simulink model "trackingModel"  (R2020b)
settings: Solver=VariableStepAuto  StartTime=0.0  StopTime=1.0  FixedStep=(1/16367600)/3  RelTol=1e-3
values from neighbouring files (symbols this model uses):
  fcBasis = 4128460    [config.m]
  fs = 16367600    [config.m]
  svnum = 22    [config.m]
libraries: commfilt2 x6, simulink x1, dspsrcs4 x1, simulink_extras x1, dspsigops x1
settings Model: Creator=sanke  LastModifiedBy=sanke
settings OptimizationCC: BlockReduction=off  ConditionallyExecuteInputs=off  DefaultParameterBehavior=Inlined
settings DebuggingCC: SignalInfNanChecking=error  AlgebraicLoopMsg=error
settings HardwareCC: ProdBitPerPointer=32  ProdBitPerSizeT=32  ProdBitPerPtrDiffT=32  ProdLargestAtomicFloat=None  ProdIntDivRoundTo=Undefined  ProdEndianess=Unspecified  ProdWordSize=32  ProdHWDeviceType=ASIC/FPGA->ASIC/FPGA  TargetBitPerPointer=64  TargetBitPerSizeT=64  TargetBitPerPtrDiffT=64  TargetLongLongMode=on  TargetIntDivRoundTo=Zero  TargetEndianess=LittleEndian  TargetWordSize=64  TargetHWDeviceType=Custom Processor->MATLAB Host Computer  ProdEqTarget=off

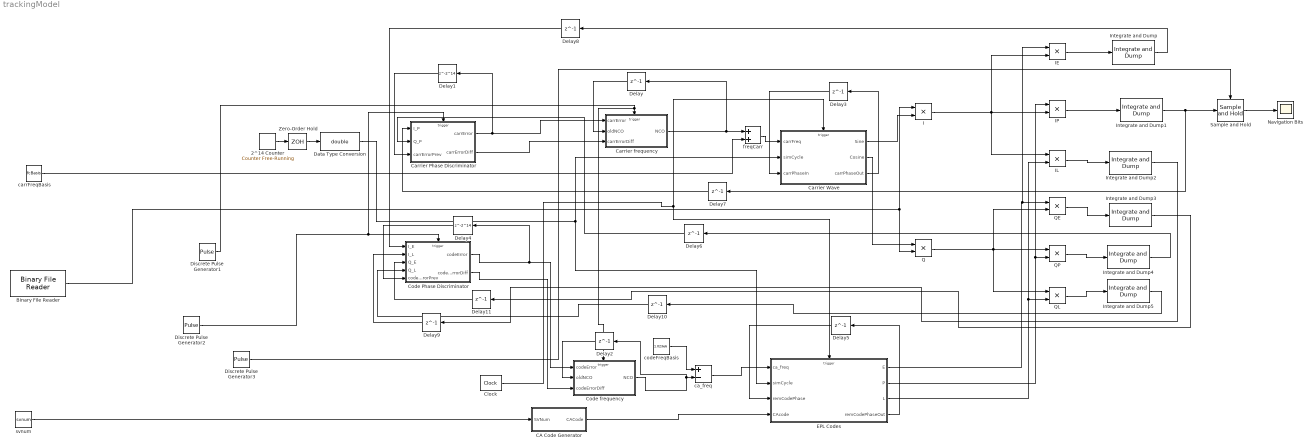
== system trackingModel ==
  2^14 Counter : simulink/Sources/Counter Free-Running  NumBits=14  tsamp=1/fs
  Binary File Reader : dspsrcs4/Binary File Reader  Filename=C:\Users\sanke\Documents\DigitalCorrelator\OscData\sv22.bin  HeaderStructure=struct([])  DataType=int8  SamplesPerFrame=1  IsDataComplex=off  NumChannels=1  OutputEOF=off  SampleTime=1/fs  SimulateUsing=Code generation
      settings: SourceProductBaseCode=DS
  CA Code Generator : Subsystem  TreatAsAtomicUnit=on
  Carrier Phase Discriminator : Subsystem  TreatAsAtomicUnit=on
  Carrier Wave : Subsystem  TreatAsAtomicUnit=on
  Carrier frequency : Subsystem  TreatAsAtomicUnit=on
  Clock : simulink_extras/Flip Flops/Clock  period=1/fs
  Code Phase Discriminator : Subsystem  TreatAsAtomicUnit=on
  Code frequency : Subsystem  TreatAsAtomicUnit=on
  Data Type Conversion : DataTypeConversion  OutDataTypeStr=double
  Delay{,2..3,5..11} (10 alike) : Delay  DelayLength=1  InitialCondition=0  SampleTime=1/fs
  Delay1 : Delay  DelayLength=2^14  InitialCondition=0  SampleTime=1/fs
  Delay4 : Delay  DelayLength=2^14  InitialCondition=0  SampleTime=1/fs
  Discrete Pulse Generator1 : DiscretePulseGenerator  Period=2^14  PulseWidth=5  PhaseDelay=2^14  SampleTime=1/fs
  Discrete Pulse Generator2 : DiscretePulseGenerator  Period=2^14  PulseWidth=5  PhaseDelay=2^14-20  SampleTime=1/fs
  Discrete Pulse Generator3 : DiscretePulseGenerator  Period=2^14  PulseWidth=5  PhaseDelay=2^14-2  SampleTime=1/fs
  EPL Codes : Subsystem  TreatAsAtomicUnit=on
  I : Product
  IE : Product
  IL : Product
  IP : Product
  Integrate and Dump{,1..5} (6 alike) : commfilt2/Integrate and Dump  obssamples=2^14  offsetsamples=0  nodump=on  roundingMode=Floor  overflowMode=off  outputDataTypeStr=Inherit: Same as accumulator  outputLastDataTypeStr=Inherit: Same as accumulator
  Navigation Bits : Scope
  Q : Product
  QE : Product
  QL : Product
  QP : Product
  Sample and Hold : dspsigops/Sample and Hold  trig=Rising edge  initCond=0  latchinput=off
  Zero-Order Hold : ZeroOrderHold  SampleTime=1/fs
  ca_freq : Sum  Inputs=+-
  carrFreqBasis : Constant  Value=fcBasis
  codeFreqBasis : Constant  Value=1.023e6
  freqCarr : Sum
  svnum : Constant  Value=svnum
  wires:
  carrFreqBasis/1 -> freqCarr/2
  freqCarr/1 -> Carrier Wave/1(carrFreq)
  Carrier Phase Discriminator/1(carrError) -> Carrier frequency/1(carrError), Delay1/1
  Carrier Phase Discriminator/2(carrErrorDiff) -> Carrier frequency/3(carrErrorDiff)
  Delay/1 -> Carrier frequency/2(oldNCO)
  Delay1/1 -> Carrier Phase Discriminator/3(carrErrorPrev)
  Carrier Wave/3(carrPhaseOut) -> Delay3/1
  Delay3/1 -> Carrier Wave/3(carrPhaseIn)
  2^14 Counter/1 -> Zero-Order Hold/1
  Zero-Order Hold/1 -> Data Type Conversion/1
  Carrier Wave/1(Sine) -> I/2
  Carrier Wave/2(Cosine) -> Q/1
  I/1 -> IL/1, IE/2, IP/2
  Q/1 -> QE/2, QL/1, QP/1
  IE/1 -> Integrate and Dump/1
  IL/1 -> Integrate and Dump2/1
  QE/1 -> Integrate and Dump3/1
  QP/1 -> Integrate and Dump4/1
  QL/1 -> Integrate and Dump5/1
  Integrate and Dump/1 -> Delay8/1
  Discrete Pulse Generator1/1 -> Code frequency/Trigger, Carrier frequency/Trigger
  Clock/1 -> EPL Codes/Trigger, Carrier Wave/Trigger
  svnum/1 -> CA Code Generator/1(SVNum)
  Data Type Conversion/1 -> Carrier Wave/2(simCycle), EPL Codes/2(simCycle)
  Binary File Reader/1 -> Q/2, I/1
  Integrate and Dump1/1 -> Delay7/1, Sample and Hold/1
  Integrate and Dump4/1 -> Delay6/1
  Integrate and Dump3/1 -> Delay11/1
  Integrate and Dump5/1 -> Delay10/1
  Integrate and Dump2/1 -> Delay9/1
  codeFreqBasis/1 -> ca_freq/1
  ca_freq/1 -> EPL Codes/1(ca_freq)
  CA Code Generator/1(CACode) -> EPL Codes/4(CAcode)
  Code Phase Discriminator/1(codeError) -> Delay4/1, Code frequency/1(codeError)
  Code Phase Discriminator/2(codeErrorDiff) -> Code frequency/3(codeErrorDiff)
  Code frequency/1(NCO) -> Delay2/1, ca_freq/2
  EPL Codes/1(E) -> IE/1, QE/1
  EPL Codes/2(P) -> IP/1, QP/2
  EPL Codes/3(L) -> IL/2, QL/2
  Delay2/1 -> Code frequency/2(oldNCO)
  Delay4/1 -> Code Phase Discriminator/5(codeErrorPrev)
  Carrier frequency/1(NCO) -> Delay/1, freqCarr/1
  Delay7/1 -> Carrier Phase Discriminator/1(I_P)
  Delay6/1 -> Carrier Phase Discriminator/2(Q_P)
  Delay8/1 -> Code Phase Discriminator/1(I_E)
  Delay9/1 -> Code Phase Discriminator/2(I_L)
  Delay11/1 -> Code Phase Discriminator/3(Q_E)
  Delay10/1 -> Code Phase Discriminator/4(Q_L)
  IP/1 -> Integrate and Dump1/1
  EPL Codes/4(remCodePhaseOut) -> Delay5/1
  Delay5/1 -> EPL Codes/3(remCodePhase)
  Sample and Hold/1 -> Navigation Bits/1
  Discrete Pulse Generator2/1 -> Carrier Phase Discriminator/Trigger, Code Phase Discriminator/Trigger
  Discrete Pulse Generator3/1 -> Sample and Hold/Trigger

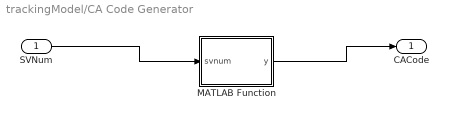
== system trackingModel/CA Code Generator ==
  SVNum : Inport
  MATLAB Function : MATLAB Function  TreatAsAtomicUnit=on
  CACode : Outport
  wires:
  SVNum/1 -> MATLAB Function/1(svnum)
  MATLAB Function/1(y) -> CACode/1

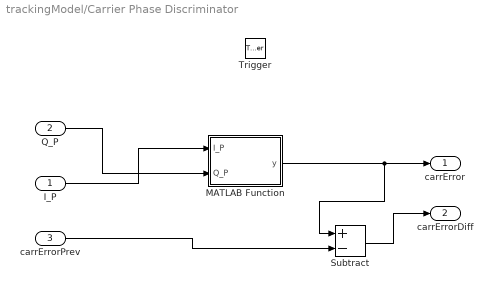
== system trackingModel/Carrier Phase Discriminator ==
  I_P : Inport
  Q_P : Inport  Port=2
  carrErrorPrev : Inport  Port=3
  Trigger : TriggerPort  VariantControl=Variant  InitialTriggerSignalState=zero
  MATLAB Function : MATLAB Function  TreatAsAtomicUnit=on
  Subtract : Sum  Inputs=+-
  carrError : Outport  InitialOutput=0
  carrErrorDiff : Outport  Port=2  InitialOutput=0
  wires:
  MATLAB Function/1(y) -> Subtract/1, carrError/1
  carrErrorPrev/1 -> Subtract/2
  Subtract/1 -> carrErrorDiff/1
  I_P/1 -> MATLAB Function/1(I_P)
  Q_P/1 -> MATLAB Function/2(Q_P)

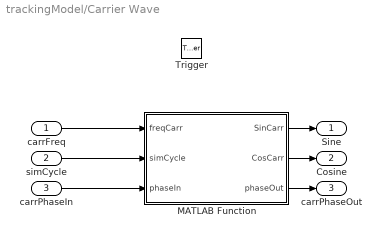
== system trackingModel/Carrier Wave ==
  carrFreq : Inport
  simCycle : Inport  Port=2
  carrPhaseIn : Inport  Port=3
  Trigger : TriggerPort  VariantControl=Variant  InitialTriggerSignalState=zero
  MATLAB Function : MATLAB Function  TreatAsAtomicUnit=on
  Sine : Outport  InitialOutput=0
  Cosine : Outport  Port=2  InitialOutput=0
  carrPhaseOut : Outport  Port=3  InitialOutput=0
  wires:
  MATLAB Function/1(SinCarr) -> Sine/1
  carrFreq/1 -> MATLAB Function/1(freqCarr)
  simCycle/1 -> MATLAB Function/2(simCycle)
  carrPhaseIn/1 -> MATLAB Function/3(phaseIn)
  MATLAB Function/2(CosCarr) -> Cosine/1
  MATLAB Function/3(phaseOut) -> carrPhaseOut/1

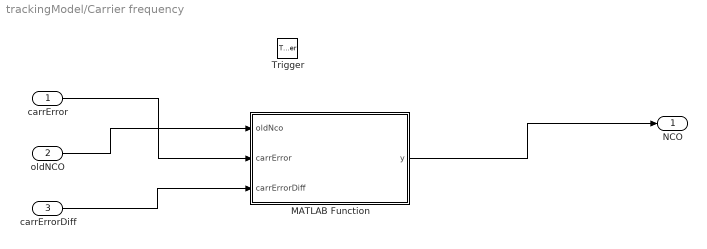
== system trackingModel/Carrier frequency ==
  carrError : Inport
  oldNCO : Inport  Port=2
  carrErrorDiff : Inport  Port=3
  Trigger : TriggerPort  VariantControl=Variant  OutputDataType=double  InitialTriggerSignalState=zero
  MATLAB Function : MATLAB Function  TreatAsAtomicUnit=on
  NCO : Outport  InitialOutput=0
  wires:
  MATLAB Function/1(y) -> NCO/1
  carrError/1 -> MATLAB Function/2(carrError)
  oldNCO/1 -> MATLAB Function/1(oldNco)
  carrErrorDiff/1 -> MATLAB Function/3(carrErrorDiff)

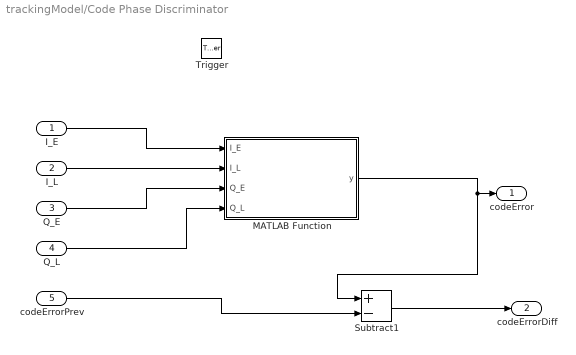
== system trackingModel/Code Phase Discriminator ==
  I_E : Inport
  I_L : Inport  Port=2
  Q_E : Inport  Port=3
  Q_L : Inport  Port=4
  codeErrorPrev : Inport  Port=5
  Trigger : TriggerPort  VariantControl=Variant  InitialTriggerSignalState=zero
  MATLAB Function : MATLAB Function  TreatAsAtomicUnit=on
  Subtract1 : Sum  Inputs=+-
  codeError : Outport  InitialOutput=0
  codeErrorDiff : Outport  Port=2  InitialOutput=0
  wires:
  MATLAB Function/1(y) -> Subtract1/1, codeError/1
  codeErrorPrev/1 -> Subtract1/2
  Subtract1/1 -> codeErrorDiff/1
  I_E/1 -> MATLAB Function/1(I_E)
  I_L/1 -> MATLAB Function/2(I_L)
  Q_E/1 -> MATLAB Function/3(Q_E)
  Q_L/1 -> MATLAB Function/4(Q_L)

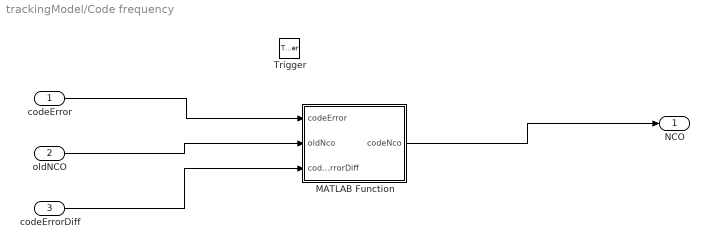
== system trackingModel/Code frequency ==
  codeError : Inport
  oldNCO : Inport  Port=2
  codeErrorDiff : Inport  Port=3
  Trigger : TriggerPort  VariantControl=Variant  OutputDataType=double  InitialTriggerSignalState=zero
  MATLAB Function : MATLAB Function  TreatAsAtomicUnit=on
  NCO : Outport  InitialOutput=0
  wires:
  MATLAB Function/1(codeNco) -> NCO/1
  codeError/1 -> MATLAB Function/1(codeError)
  oldNCO/1 -> MATLAB Function/2(oldNco)
  codeErrorDiff/1 -> MATLAB Function/3(codeErrorDiff)

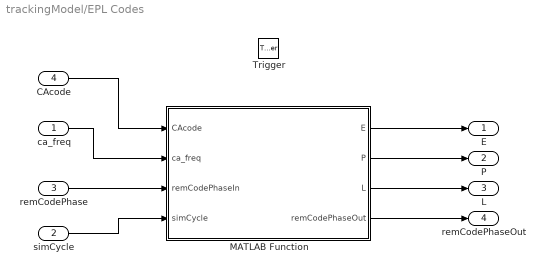
== system trackingModel/EPL Codes ==
  ca_freq : Inport
  simCycle : Inport  Port=2
  remCodePhase : Inport  Port=3
  CAcode : Inport  Port=4
  Trigger : TriggerPort  VariantControl=Variant  InitialTriggerSignalState=zero
  MATLAB Function : MATLAB Function  TreatAsAtomicUnit=on
  E : Outport  InitialOutput=0
  P : Outport  Port=2  InitialOutput=0
  L : Outport  Port=3  InitialOutput=0
  remCodePhaseOut : Outport  Port=4  InitialOutput=0
  wires:
  CAcode/1 -> MATLAB Function/1(CAcode)
  ca_freq/1 -> MATLAB Function/2(ca_freq)
  remCodePhase/1 -> MATLAB Function/3(remCodePhaseIn)
  simCycle/1 -> MATLAB Function/4(simCycle)
  MATLAB Function/1(E) -> E/1
  MATLAB Function/2(P) -> P/1
  MATLAB Function/3(L) -> L/1
  MATLAB Function/4(remCodePhaseOut) -> remCodePhaseOut/1

== matlab function trackingModel/CA Code Generator/MATLAB Function ==
  data: svnum input; y output
function y = CAGen(svnum)
g2s = [5;6;7;8;17;18;139;140;141;251;252;254;255;256;257;258; 469;470;471; ...
     472;473;474;509;512;513;514;515;516;859;860;861;862]; 
 
g2shift = g2s(svnum,1);

% Generate G1 code
% load shift register 
reg = -1*ones(1,10);
g1 = zeros(1,1023);
for i = 1:1023
    g1(i) = reg(10);
    save1 = reg(3)*reg(10); 
    reg(1,2:10) = reg(1:1:9); 
    reg(1) = save1;
end

%  Generate G2 code 
% load shift register 
reg = -1*ones(1,10);
g2 = zeros(1,1023);
for i = 1:1023
    g2(i) = reg(10);
    save2 = reg(2)*reg(3)*reg(6)*reg(8)*reg(9)*reg(10);
    reg(1,2:10) = reg(1:1:9);
    reg(1) = save2; 
end

% Shift G2 code
g2tmp = zeros(1,1023);
g2tmp(1,1:g2shift) = g2(1,1023-g2shift+1:1023); 
g2tmp(1,g2shift+1:1023) = g2(1,1:1023-g2shift); 
g2 = g2tmp;
%
% Form single sample C/A code by multiplying G1 and G2 %
ss_ca = g1.*g2;
y = -ss_ca;

== matlab function trackingModel/Carrier Wave/MATLAB Function ==
  data: freqCarr input; SinCarr output; simCycle input; phaseIn input; CosCarr output; phaseOut output
function [SinCarr, CosCarr, phaseOut] = fcn(freqCarr, simCycle, phaseIn)

SinCarr = sin(freqCarr*2*pi*simCycle/16367600 + phaseIn);
CosCarr = cos(freqCarr*2*pi*simCycle/16367600 + phaseIn);
if simCycle < 2^14 - 1
    phaseOut = phaseIn;
else
    phaseOut = rem(freqCarr*2*pi*2^14/16367600+phaseIn, 2*pi);
end

== matlab function trackingModel/EPL Codes/MATLAB Function ==
  data: CAcode input; E output; ca_freq input; remCodePhaseIn input; simCycle input; P output; L output; remCodePhaseOut output
function [E, P, L, remCodePhaseOut] = EPLGenerator(CAcode, ca_freq, remCodePhaseIn, simCycle)

CAcode = [CAcode(1023) CAcode CAcode];

%Early
tcode = ceil(remCodePhaseIn-0.5+simCycle*ca_freq/16367600)+1;
E = CAcode(tcode);

%Late
tcode = ceil(remCodePhaseIn+0.5+simCycle*ca_freq/16367600)+1;
L = CAcode(tcode);

%Prompt
tcode = ceil(remCodePhaseIn+simCycle*ca_freq/16367600)+1;
P = CAcode(tcode);

if simCycle < 2^14 - 1
    remCodePhaseOut = remCodePhaseIn;
else
    remCodePhaseOut = remCodePhaseIn+2^14*ca_freq/16367600 - 1023.0;
end

== matlab function trackingModel/Code Phase Discriminator/MATLAB Function ==
  data: I_E input; y output; I_L input; Q_E input; Q_L input
function y = codeError(I_E, I_L, Q_E, Q_L)


if I_E~=0 || I_L~=0 || Q_E~= 0 || Q_L ~= 0
    y = (sqrt(I_E * I_E + Q_E * Q_E) - sqrt(I_L * I_L + Q_L * Q_L)) / ...
                (sqrt(I_E * I_E + Q_E * Q_E) + sqrt(I_L * I_L + Q_L * Q_L));
else
    y=0;
end

== matlab function trackingModel/Carrier Phase Discriminator/MATLAB Function ==
  data: I_P input; y output; Q_P input
function y = carrError(I_P, Q_P)

if I_P~=0 || Q_P~= 0
    y = atan(Q_P / I_P) / (2.0 * pi);
else
    y=0;
end

== matlab function trackingModel/Code frequency/MATLAB Function ==
  data: codeError input; codeNco output; oldNco input; codeErrorDiff input
function codeNco  = fcn(codeError, oldNco, codeErrorDiff)

tau1code = 0.011175510204082;
tau2code = 0.148;
PDIcode = 0;

codeNco = oldNco + (tau2code/tau1code) * (codeErrorDiff) + codeError * (PDIcode/tau1code);

== matlab function trackingModel/Carrier frequency/MATLAB Function ==
  data: oldNco input; y output; carrError input; carrErrorDiff input
function y = carrNco(oldNco, carrError, carrErrorDiff)

tau1carr = 1.117551020408163e-04;
tau2carr = 0.0296;
PDIcarr = 0;

y = oldNco + (tau2carr/tau1carr) * (carrErrorDiff) + carrError * (PDIcarr/tau1carr);
